simulink model "fohdemo"  (Simulink 6.0)
settings: Solver=VariableStepDiscrete  SolverMode=SingleTasking  StartTime=0.0  StopTime=3  MaxStep=.01  RelTol=1e-3  AbsTol=1e-6
libraries: simulink x1
settings Model: Creator=The MathWorks Inc.  LastModifiedBy=batserve  ExtModeTrigMode=oneshot  ExtModeArmWhenConnect=off  ExtModeAutoUpdateStatusClock=off
settings DataIOCC: ExternalInput=[]  InitialState=[]  LimitDataPoints=off  SaveOutput=off  TimeSaveName=t
settings OptimizationCC: BooleanDataType=off
settings DebuggingCC: CheckExecutionContextPreStartOutputMsg=on  CheckExecutionContextRuntimeOutputMsg=on  SolverPrmCheckMsg=none  IntegerOverflowMsg=none
settings HardwareCC: TargetUnknown=on

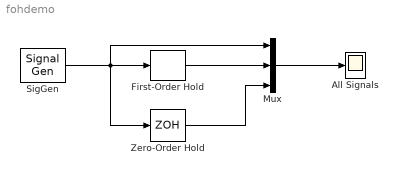
== system fohdemo ==
  All Signals : Scope
      settings: TickLabels=on  TimeRange=3  DataFormat=Array
  First-Order Hold : simulink/Discrete/First-Order Hold  DisableCoverage=on  Ts=0.1
  Mux : Mux  Inputs=3
  SigGen : SignalGenerator  Amplitude=5.000000  Frequency=1.000000
  Zero-Order Hold : ZeroOrderHold  SampleTime=0.1
  wires:
  SigGen/1 -> Mux/1, Zero-Order Hold/1, First-Order Hold/1
  Zero-Order Hold/1 -> Mux/3
  First-Order Hold/1 -> Mux/2
  Mux/1 -> All Signals/1
